simulink model "controller_joint"  (R2020a)
settings: Solver=ode3  StartTime=0.0  StopTime=inf  FixedStep=0.05  RelTol=1e-3
libraries: robotlib x35, robotmaniplib x1
settings Model: Creator=paolo  LastModifiedBy=paolo
settings OptimizationCC: EnhancedBackFolding=on  PassReuseOutputArgsAs=Individual arguments  ZeroExternalMemoryAtStartup=off  ZeroInternalMemoryAtStartup=off  MaxStackSize=64  OptimizeBlockOrder=speed  DifferentSizesBufferReuse=on  OptimizationCustomize=off  EfficientTunableParamExpr=on
settings DebuggingCC: ParameterTunabilityLossMsg=error
settings HardwareCC: ProdBitPerPointer=32  ProdBitPerSizeT=32  ProdBitPerPtrDiffT=32  ProdLargestAtomicFloat=None  ProdIntDivRoundTo=Undefined  ProdEndianess=Unspecified  ProdWordSize=32  ProdHWDeviceType=Generic->Unspecified (assume 32-bit Generic)
settings SFSimCC: MATLABDynamicMemAlloc=off
settings RTWCC: SystemTargetFile=ert.tlc  HardwareBoard=Robot Operating System (ROS)  TemplateMakefile=ert_default_tmf  Toolchain=Catkin  TargetLang=C++
settings CodeAppCC: ForceParamTrailComments=on  IgnoreCustomStorageClasses=off  OperatorAnnotations=on  SimulinkDataObjDesc=on  SFDataObjDesc=on  InsertBlockDesc=on

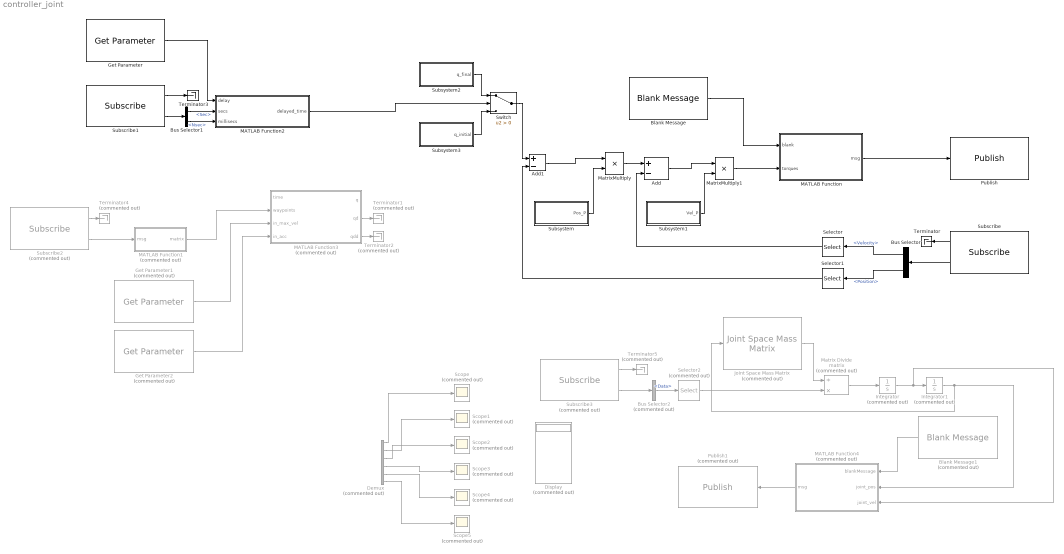
== system controller_joint ==
  Add : Sum  Inputs=+-
  Add1 : Sum  Inputs=+-
  Blank Message : robotlib/Blank Message  messageClass=Message  entityType=std_msgs/Float64MultiArray  messageType=std_msgs/Float64MultiArray  SampleTime=inf
  Blank Message1 : robotlib/Blank Message  Commented=on  messageClass=Message  entityType=sensor_msgs/JointState  messageType=sensor_msgs/JointState  SampleTime=inf
  Bus Selector : BusSelector  OutputSignals=Velocity,Position
  Bus Selector1 : BusSelector  OutputSignals=Clock_.Sec,Clock_.Nsec
  Bus Selector2 : BusSelector  Commented=on  OutputSignals=Data
  Demux : Demux  Commented=on  Outputs=6
  Display : Display  Commented=on
  Get Parameter : robotlib/Get Parameter  ParameterSource=Specify your own  ParameterName=/start_delay  ParameterType=double  ParameterMaxArrayLength=16  ParameterInitialValue=10  SampleTime=-1  ShowErrorCodeOutput=off  ModelName=controller_joint  BlockId=ParamGet_controller_joint_55
      settings: SourceProductBaseCode=RR
  Get Parameter1 : robotlib/Get Parameter  Commented=on  ParameterSource=Specify your own  ParameterName=/max_ang_vel  ParameterType=double  ParameterMaxArrayLength=16  ParameterInitialValue=1  SampleTime=-1  ShowErrorCodeOutput=off  ModelName=controller_joint  BlockId=ParamGet_controller_joint_38
      settings: SourceProductBaseCode=RR
  Get Parameter2 : robotlib/Get Parameter  Commented=on  ParameterSource=Specify your own  ParameterName=/max_ang_acc  ParameterType=double  ParameterMaxArrayLength=16  ParameterInitialValue=0.5  SampleTime=-1  ShowErrorCodeOutput=off  ModelName=controller_joint  BlockId=ParamGet_controller_joint_39
      settings: SourceProductBaseCode=RR
  Integrator : Integrator  Commented=on
  Integrator1 : Integrator  Commented=on
  Joint Space Mass Matrix : robotmaniplib/Joint Space Mass Matrix  Commented=on  RigidBodyTree=robot  SimulateUsing=Interpreted execution
  MATLAB Function : MATLAB Function  TreatAsAtomicUnit=on
  MATLAB Function1 : MATLAB Function  Commented=on  TreatAsAtomicUnit=on
  MATLAB Function2 : MATLAB Function  TreatAsAtomicUnit=on
  MATLAB Function3 : MATLAB Function  Commented=on  TreatAsAtomicUnit=on
  MATLAB Function4 : MATLAB Function  Commented=on  TreatAsAtomicUnit=on
  Matrix Divide : Product  Commented=on  Inputs=/*  Multiplication=Matrix(*)
  MatrixMultiply : Product
  MatrixMultiply1 : Product
  Publish : robotlib/Publish  topicSource=Specify your own  topic=/joint_torque  messageType=std_msgs/Float64MultiArray  messageQueueLength=1
  Publish1 : robotlib/Publish  Commented=on  topicSource=Specify your own  topic=/joint_states  messageType=sensor_msgs/JointState  messageQueueLength=1
  Scope{,1..5} (6 alike) : Scope  Commented=on
  Selector : Selector  InputPortWidth=128  IndexOptions=Starting index (dialog)  Indices=[1]  OutputSizes=6
  Selector1 : Selector  InputPortWidth=128  IndexOptions=Starting index (dialog)  Indices=1  OutputSizes=6
  Selector2 : Selector  Commented=on  IndexOptions=Starting index (dialog)  Indices=1  OutputSizes=6
  Subscribe : robotlib/Subscribe  topicSource=Specify your own  topic=/joint_states  messageType=sensor_msgs/JointState  sampleTime=-1  messageQueueLength=1
  Subscribe1 : robotlib/Subscribe  topicSource=Specify your own  topic=/clock  messageType=rosgraph_msgs/Clock  sampleTime=-1  messageQueueLength=1
  Subscribe2 : robotlib/Subscribe  Commented=on  topicSource=Specify your own  topic=/joint_waypoints  messageType=std_msgs/Float32MultiArray  sampleTime=-1  messageQueueLength=1
  Subscribe3 : robotlib/Subscribe  Commented=on  topicSource=Specify your own  topic=/joint_torque  messageType=std_msgs/Float64MultiArray  sampleTime=-1  messageQueueLength=1
  Subsystem : Subsystem
  Subsystem1 : Subsystem
  Subsystem2 : Subsystem
  Subsystem3 : Subsystem
  Switch : Switch  Criteria=u2 > Threshold
  Terminator : Terminator
  Terminator{1..2,4..5} (4 alike) : Terminator  Commented=on
  Terminator3 : Terminator
  wires:
  Add/1 -> MatrixMultiply1/1
  MatrixMultiply/1 -> Add/1
  MatrixMultiply1/1 -> MATLAB Function/2(torques)
  Blank Message/1 -> MATLAB Function/1(blank)
  MATLAB Function/1(msg) -> Publish/1
  Subscribe/1 -> Terminator/1
  Subscribe/2 -> Bus Selector/1
  Selector/1 -> Add/2
  Selector1/1 -> Add1/2
  Subscribe1/1 -> Terminator3/1
  Subscribe1/2 -> Bus Selector1/1
  Bus Selector1/1 -> MATLAB Function2/2(secs)  "<Sec>"
  Bus Selector1/2 -> MATLAB Function2/3(millisecs)  "<Nsec>"
  Get Parameter/1 -> MATLAB Function2/1(delay)
  Subscribe2/2 -> MATLAB Function1/1(msg)
  MATLAB Function1/1(matrix) -> MATLAB Function3/2(waypoints)
  Get Parameter2/1 -> MATLAB Function3/4(in_acc)
  Get Parameter1/1 -> MATLAB Function3/3(in_max_vel)
  MATLAB Function3/2(qd) -> Terminator1/1
  MATLAB Function3/3(qdd) -> Terminator2/1
  Bus Selector/1 -> Selector/1  "<Velocity>"
  Bus Selector/2 -> Selector1/1  "<Position>"
  Subscribe2/1 -> Terminator4/1
  Blank Message1/1 -> MATLAB Function4/1(blankMessage)
  Selector2/1 -> Matrix Divide/2
  MATLAB Function4/1(msg) -> Publish1/1
  Subscribe3/2 -> Bus Selector2/1
  Integrator/1 -> Integrator1/1, MATLAB Function4/3(joint_vel)
  Matrix Divide/1 -> Integrator/1
  Bus Selector2/1 -> Selector2/1  "<Data>"
  Integrator1/1 -> Joint Space Mass Matrix/1, MATLAB Function4/2(joint_pos)
  Joint Space Mass Matrix/1 -> Matrix Divide/1
  Subscribe3/1 -> Terminator5/1
  Demux/2 -> Scope1/1
  Demux/3 -> Scope2/1
  Demux/4 -> Scope3/1
  Demux/5 -> Scope4/1
  Demux/6 -> Scope5/1
  Demux/1 -> Scope/1
  Add1/1 -> MatrixMultiply/1
  Subsystem/1(Pos_P) -> MatrixMultiply/2
  Subsystem1/1(Vel_P) -> MatrixMultiply1/2
  Subsystem3/1(q_initial) -> Switch/3
  Subsystem2/1(q_final) -> Switch/1
  Switch/1 -> Add1/1
  MATLAB Function2/1(delayed_time) -> Switch/2

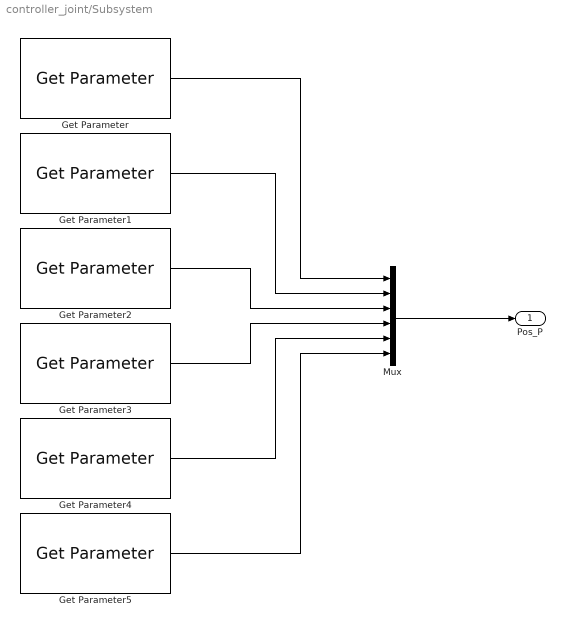
== system controller_joint/Subsystem ==
  Get Parameter : robotlib/Get Parameter  ParameterSource=Specify your own  ParameterName=/pos_control_1  ParameterType=double  ParameterMaxArrayLength=16  ParameterInitialValue=0.1  SampleTime=-1  ShowErrorCodeOutput=off  ModelName=controller_joint  BlockId=ParamGet_controller_joint_93
      settings: SourceProductBaseCode=RR
  Get Parameter1 : robotlib/Get Parameter  ParameterSource=Specify your own  ParameterName=/pos_control_2  ParameterType=double  ParameterMaxArrayLength=16  ParameterInitialValue=0.1  SampleTime=-1  ShowErrorCodeOutput=off  ModelName=controller_joint  BlockId=ParamGet_controller_joint_94
      settings: SourceProductBaseCode=RR
  Get Parameter2 : robotlib/Get Parameter  ParameterSource=Specify your own  ParameterName=/pos_control_3  ParameterType=double  ParameterMaxArrayLength=16  ParameterInitialValue=0.1  SampleTime=-1  ShowErrorCodeOutput=off  ModelName=controller_joint  BlockId=ParamGet_controller_joint_95
      settings: SourceProductBaseCode=RR
  Get Parameter3 : robotlib/Get Parameter  ParameterSource=Specify your own  ParameterName=/pos_control_4  ParameterType=double  ParameterMaxArrayLength=16  ParameterInitialValue=0.1  SampleTime=-1  ShowErrorCodeOutput=off  ModelName=controller_joint  BlockId=ParamGet_controller_joint_96
      settings: SourceProductBaseCode=RR
  Get Parameter4 : robotlib/Get Parameter  ParameterSource=Specify your own  ParameterName=/pos_control_5  ParameterType=double  ParameterMaxArrayLength=16  ParameterInitialValue=0.1  SampleTime=-1  ShowErrorCodeOutput=off  ModelName=controller_joint  BlockId=ParamGet_controller_joint_97
      settings: SourceProductBaseCode=RR
  Get Parameter5 : robotlib/Get Parameter  ParameterSource=Specify your own  ParameterName=/pos_control_6  ParameterType=double  ParameterMaxArrayLength=16  ParameterInitialValue=0.1  SampleTime=-1  ShowErrorCodeOutput=off  ModelName=controller_joint  BlockId=ParamGet_controller_joint_98
      settings: SourceProductBaseCode=RR
  Mux : Mux  Inputs=6
  Pos_P : Outport
  wires:
  Mux/1 -> Pos_P/1
  Get Parameter/1 -> Mux/1
  Get Parameter1/1 -> Mux/2
  Get Parameter2/1 -> Mux/3
  Get Parameter3/1 -> Mux/4
  Get Parameter4/1 -> Mux/5
  Get Parameter5/1 -> Mux/6

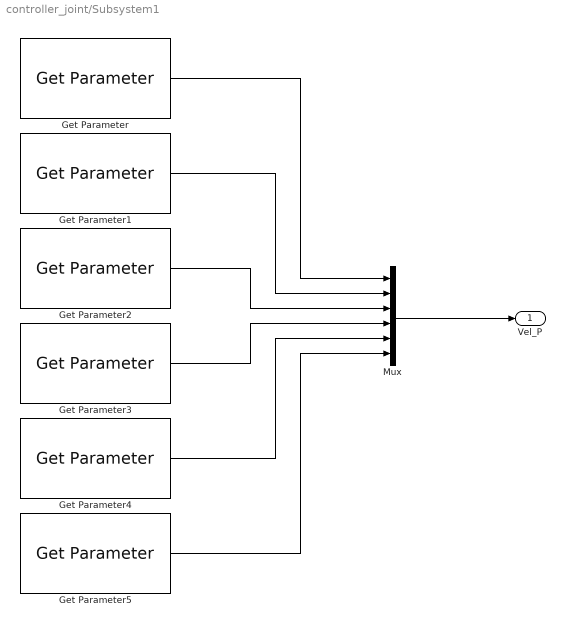
== system controller_joint/Subsystem1 ==
  Get Parameter : robotlib/Get Parameter  ParameterSource=Specify your own  ParameterName=/vel_control_1  ParameterType=double  ParameterMaxArrayLength=16  ParameterInitialValue=0.1  SampleTime=-1  ShowErrorCodeOutput=off  ModelName=controller_joint  BlockId=ParamGet_controller_joint_103
      settings: SourceProductBaseCode=RR
  Get Parameter1 : robotlib/Get Parameter  ParameterSource=Specify your own  ParameterName=/vel_control_2  ParameterType=double  ParameterMaxArrayLength=16  ParameterInitialValue=0.1  SampleTime=-1  ShowErrorCodeOutput=off  ModelName=controller_joint  BlockId=ParamGet_controller_joint_104
      settings: SourceProductBaseCode=RR
  Get Parameter2 : robotlib/Get Parameter  ParameterSource=Specify your own  ParameterName=/vel_control_3  ParameterType=double  ParameterMaxArrayLength=16  ParameterInitialValue=0.1  SampleTime=-1  ShowErrorCodeOutput=off  ModelName=controller_joint  BlockId=ParamGet_controller_joint_105
      settings: SourceProductBaseCode=RR
  Get Parameter3 : robotlib/Get Parameter  ParameterSource=Specify your own  ParameterName=/vel_control_4  ParameterType=double  ParameterMaxArrayLength=16  ParameterInitialValue=0.01  SampleTime=-1  ShowErrorCodeOutput=off  ModelName=controller_joint  BlockId=ParamGet_controller_joint_106
      settings: SourceProductBaseCode=RR
  Get Parameter4 : robotlib/Get Parameter  ParameterSource=Specify your own  ParameterName=/vel_control_5  ParameterType=double  ParameterMaxArrayLength=16  ParameterInitialValue=0.1  SampleTime=-1  ShowErrorCodeOutput=off  ModelName=controller_joint  BlockId=ParamGet_controller_joint_107
      settings: SourceProductBaseCode=RR
  Get Parameter5 : robotlib/Get Parameter  ParameterSource=Specify your own  ParameterName=/vel_control_6  ParameterType=double  ParameterMaxArrayLength=16  ParameterInitialValue=1e-4  SampleTime=-1  ShowErrorCodeOutput=off  ModelName=controller_joint  BlockId=ParamGet_controller_joint_108
      settings: SourceProductBaseCode=RR
  Mux : Mux  Inputs=6
  Vel_P : Outport
  wires:
  Get Parameter4/1 -> Mux/5
  Mux/1 -> Vel_P/1
  Get Parameter/1 -> Mux/1
  Get Parameter5/1 -> Mux/6
  Get Parameter2/1 -> Mux/3
  Get Parameter3/1 -> Mux/4
  Get Parameter1/1 -> Mux/2

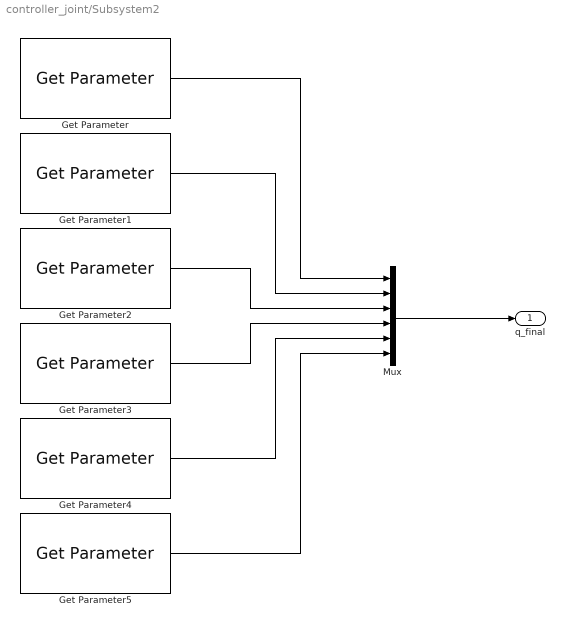
== system controller_joint/Subsystem2 ==
  Get Parameter : robotlib/Get Parameter  ParameterSource=Specify your own  ParameterName=/q1_final  ParameterType=double  ParameterMaxArrayLength=16  ParameterInitialValue=1.57  SampleTime=-1  ShowErrorCodeOutput=off  ModelName=controller_joint  BlockId=ParamGet_controller_joint_115
      settings: SourceProductBaseCode=RR
  Get Parameter1 : robotlib/Get Parameter  ParameterSource=Specify your own  ParameterName=/q2_final  ParameterType=double  ParameterMaxArrayLength=16  ParameterInitialValue=1.57  SampleTime=-1  ShowErrorCodeOutput=off  ModelName=controller_joint  BlockId=ParamGet_controller_joint_116
      settings: SourceProductBaseCode=RR
  Get Parameter2 : robotlib/Get Parameter  ParameterSource=Specify your own  ParameterName=/q3_final  ParameterType=double  ParameterMaxArrayLength=16  ParameterInitialValue=1.57  SampleTime=-1  ShowErrorCodeOutput=off  ModelName=controller_joint  BlockId=ParamGet_controller_joint_117
      settings: SourceProductBaseCode=RR
  Get Parameter3 : robotlib/Get Parameter  ParameterSource=Specify your own  ParameterName=/q4_final  ParameterType=double  ParameterMaxArrayLength=16  ParameterInitialValue=1.57  SampleTime=-1  ShowErrorCodeOutput=off  ModelName=controller_joint  BlockId=ParamGet_controller_joint_118
      settings: SourceProductBaseCode=RR
  Get Parameter4 : robotlib/Get Parameter  ParameterSource=Specify your own  ParameterName=/q5_final  ParameterType=double  ParameterMaxArrayLength=16  ParameterInitialValue=1.57  SampleTime=-1  ShowErrorCodeOutput=off  ModelName=controller_joint  BlockId=ParamGet_controller_joint_119
      settings: SourceProductBaseCode=RR
  Get Parameter5 : robotlib/Get Parameter  ParameterSource=Specify your own  ParameterName=/q6_final  ParameterType=double  ParameterMaxArrayLength=16  ParameterInitialValue=1.57  SampleTime=-1  ShowErrorCodeOutput=off  ModelName=controller_joint  BlockId=ParamGet_controller_joint_120
      settings: SourceProductBaseCode=RR
  Mux : Mux  Inputs=6
  q_final : Outport
  wires:
  Get Parameter4/1 -> Mux/5
  Mux/1 -> q_final/1
  Get Parameter/1 -> Mux/1
  Get Parameter5/1 -> Mux/6
  Get Parameter2/1 -> Mux/3
  Get Parameter3/1 -> Mux/4
  Get Parameter1/1 -> Mux/2

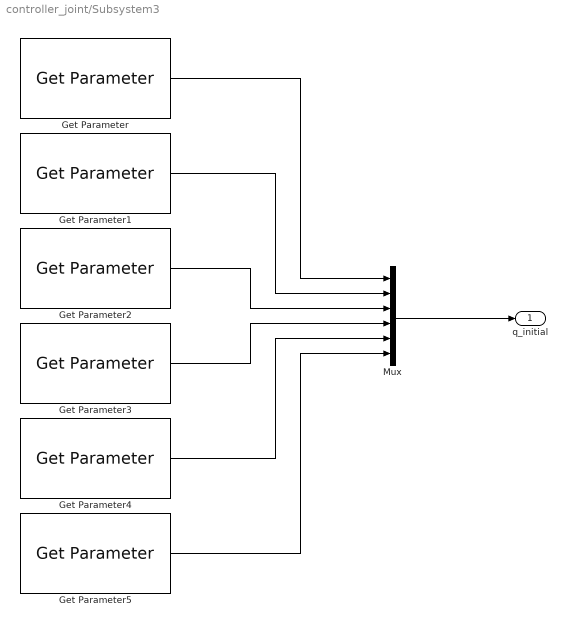
== system controller_joint/Subsystem3 ==
  Get Parameter : robotlib/Get Parameter  ParameterSource=Specify your own  ParameterName=/q1_initial  ParameterType=double  ParameterMaxArrayLength=16  ParameterInitialValue=0  SampleTime=-1  ShowErrorCodeOutput=off  ModelName=controller_joint  BlockId=ParamGet_controller_joint_127
      settings: SourceProductBaseCode=RR
  Get Parameter1 : robotlib/Get Parameter  ParameterSource=Specify your own  ParameterName=/q2_initial  ParameterType=double  ParameterMaxArrayLength=16  ParameterInitialValue=0  SampleTime=-1  ShowErrorCodeOutput=off  ModelName=controller_joint  BlockId=ParamGet_controller_joint_128
      settings: SourceProductBaseCode=RR
  Get Parameter2 : robotlib/Get Parameter  ParameterSource=Specify your own  ParameterName=/q3_initial  ParameterType=double  ParameterMaxArrayLength=16  ParameterInitialValue=0  SampleTime=-1  ShowErrorCodeOutput=off  ModelName=controller_joint  BlockId=ParamGet_controller_joint_129
      settings: SourceProductBaseCode=RR
  Get Parameter3 : robotlib/Get Parameter  ParameterSource=Specify your own  ParameterName=/q4_initial  ParameterType=double  ParameterMaxArrayLength=16  ParameterInitialValue=0  SampleTime=-1  ShowErrorCodeOutput=off  ModelName=controller_joint  BlockId=ParamGet_controller_joint_130
      settings: SourceProductBaseCode=RR
  Get Parameter4 : robotlib/Get Parameter  ParameterSource=Specify your own  ParameterName=/q5_initial  ParameterType=double  ParameterMaxArrayLength=16  ParameterInitialValue=0  SampleTime=-1  ShowErrorCodeOutput=off  ModelName=controller_joint  BlockId=ParamGet_controller_joint_131
      settings: SourceProductBaseCode=RR
  Get Parameter5 : robotlib/Get Parameter  ParameterSource=Specify your own  ParameterName=/q6_initial  ParameterType=double  ParameterMaxArrayLength=16  ParameterInitialValue=0  SampleTime=-1  ShowErrorCodeOutput=off  ModelName=controller_joint  BlockId=ParamGet_controller_joint_132
      settings: SourceProductBaseCode=RR
  Mux : Mux  Inputs=6
  q_initial : Outport
  wires:
  Get Parameter4/1 -> Mux/5
  Mux/1 -> q_initial/1
  Get Parameter/1 -> Mux/1
  Get Parameter5/1 -> Mux/6
  Get Parameter2/1 -> Mux/3
  Get Parameter3/1 -> Mux/4
  Get Parameter1/1 -> Mux/2

== matlab function controller_joint/MATLAB Function1 ==
  data: msg input; matrix output
function matrix = fcn(msg)

    matrix = zeros(6, 20);

    for i=1:6
        for j=1:20
            matrix(i, j) = msg.Data((i-1)*20+j);
        end
    end

== matlab function controller_joint/MATLAB Function ==
  data: blank input; msg output Bus: SL_Bus_controller_joint_std_msgs_Float64MultiArray; torques input
function msg = assign_message(blank, torques)

    msg = blank;
    num_joints = length(torques);

    for i=1:num_joints
        msg.Data(i) = torques(i);
    end

    msg.Data_SL_Info.CurrentLength = uint32(num_joints);

    msg.Layout.Dim_SL_Info.CurrentLength = uint32(1);

    msg.Layout.Dim(1).Size = uint32(num_joints);
    msg.Layout.Dim(1).Stride = uint32(num_joints);

== matlab function controller_joint/MATLAB Function2 ==
  data: delay input; secs input; millisecs input; delayed_time output
function delayed_time = get_time(delay, secs, millisecs)

    time = secs + millisecs / 1e9;
    delayed_time = time - delay;
    
    if delayed_time < 0
        delayed_time = 0;
    end

== matlab function controller_joint/MATLAB Function3 ==
  data: time input; q output; waypoints input; in_max_vel input; in_acc input; qd output; qdd output
function [q, qd, qdd] = fcn(time, waypoints, in_max_vel, in_acc)

q_len = length(waypoints);

q = waypoints(:, 1);
qd = zeros(q_len, 1);
qdd = zeros(q_len, 1);

[rows, columns] = size(waypoints);

if length(in_max_vel) == 1
    max_vel = in_max_vel * ones(q_len, 1);
else
    max_vel = in_max_vel;
end

if length(in_acc) == 1
    acc = in_acc * ones(q_len, 1);
else
    acc = in_acc;
end

act_max_vel = zeros(rows, columns-1);
signes = zeros(rows, columns-1);
t = zeros(rows, columns-1, 3);

for i=1:rows
    
    t_up = max_vel(i) / acc(i);
   
    for j=1:columns-1
        
        dist = waypoints(i, j+1) - waypoints(i, j);
        signes(i, j) = sign(dist);
        
        if abs(dist) < t_up * max_vel(i)
            act_t_up = sqrt(abs(dist)/acc(i));
            t(i, j, 2) = 0;
            t(i, j, 1) = act_t_up;
            t(i, j, 3) = act_t_up;
            act_max_vel(i, j) = act_t_up * acc(i);
        else
            t(i, j, 1) = t_up;
            t(i, j, 3) = t_up;
            t(i, j, 2) = (abs(dist) - t_up * max_vel(i)) / max_vel(i);
            act_max_vel(i, j) = max_vel(i);
        end
        
    end
         
end

for i=1:rows
    
    t1 = time;
    
    for j=1:columns-1
        
        if t1 <= 0
            break   
        end
        
        for k=1:3
            
            if t1 - t(i, j, k) <= 0
                if k == 1
                    q(i) = q(i) + 1/2* acc(i) * t1^2 * signes(i, j);
                    qd(i) = acc(i) * t1 * signes(i, j);
                    qdd(i) = acc(i) * signes(i, j);
                    t1 = t1 - t(i, j, k);
                    break;
                end
                if k == 2
                    q(i) = q(i) + max_vel(i) * t1 * signes(i, j);
                    qd(i) = max_vel(i) * signes(i);
                    qdd(i) = 0;
                    t1 = t1 - t(i, j, k);
                    break;
                end
                q(i) = q(i) + (act_max_vel(j) * t1 - 1/2 * acc(i) * t1^2) * signes(i, j);
                qd(i) = (act_max_vel(i) - t1 * acc(i)) * signes(i, j);
                qdd(i) = - acc(i) * signes(i, j);
                t1 = t1 - t(i, j, k);
                break;
            end
            
            t1 = t1 - t(i, j, k);
            
            if k == 1
                q(i) = q(i) + 1/2 * acc(i) * t(i, j, k)^2 * signes(i, j);
                qd(i) = act_max_vel(i) * signes(i, j);
                qdd(i) = acc(i) * signes(i, j);
            elseif k == 2
                q(i) = q(i) + max_vel(i) * t(i, j, k) * signes(i, j);
                qd(i) = act_max_vel(i) * signes(i, j);
                qdd(i) = 0;
            else
                q(i) = q(i) + (act_max_vel(i) * t(i, j, k) - 1/2 * acc(i) * t(i, j, k)^2) * signes(i, j);
                qd(i) = 0;
                qdd(i) = 0;
            end
        
        end
        
    end
    
end

== matlab function controller_joint/MATLAB Function4 ==
  data: blankMessage input; msg output Bus: SL_Bus_controller_joint_sensor_msgs_JointState; joint_pos input; joint_vel input
function msg = assign_message(blankMessage, joint_pos, joint_vel)

    msg = blankMessage;
    
    num_joints = length(joint_pos);
    
    msg.Position_SL_Info.CurrentLength = uint32(num_joints);
    msg.Velocity_SL_Info.CurrentLength = uint32(num_joints);
    
    for i=1:num_joints
        
        msg.Position(i) = joint_pos(i);
        msg.Velocity(i) = joint_vel(i);
        
    end
